simulink model "sm_rack_and_pinion_assembly_testrig"  (R2026a)
settings: Solver=ode23t  MaxStep=0.01  AbsTol=1e-4  EnableMultiTasking=on
undefined symbols (not defined in the file or in its folder): Local, Z
libraries: sm_lib x3, nesl_utility x2, Multibody_Parts_Lib x2
CloseFcn:
  | try,close(h1_sm_rack_and_pinion_assembly_testrig),end
  | clear h1_sm_rack_and_pinion_assembly_testrig
  | 
  | clear simlog_sm_rack_and_pinion_assembly_testrig
  | clear logsout_sm_rack_and_pinion_assembly_testrig
Description:
  | Rack and Pinion Assembly Testrig
  | 
  | Copyright 2014-2026 The MathWorks, Inc.
settings Model: Creator=smiller  LastModifiedBy=smiller
settings DataIOCC: SignalLoggingName=logsout_sm_rack_and_pinion_assembly_testrig
settings DebuggingCC: UnderspecifiedInitializationDetection=Classic  PregeneratedLibrarySubsystemCodeDiagnostic=none
settings HardwareCC: ProdHWDeviceType=32-bit Generic
settings SimscapeCC: SimscapeNormalizeSystem=off  SimscapeNominalValues="[{\"value\":\"1\",\"unit\":\"A\"},{\"value\":\"1\",\"unit\":\"bar\"},{\"value\":\"1\",\"unit\":\"cm^2\"},{\"value\":\"1\",\"unit\":\"cm^3/s\"},{\"value\":\"1\",\"unit\":\"kJ/kg\"},{\"value\":\"1\",\"unit\":\"kW\"},{\"value\":\"1\",\"unit\":\"l\"},{\"value\":\"1\",\"unit\":\"N\"},{\"value\":\"1\",\"unit\":\"N*m\"},{\"value\":\"1\",\"unit\":\"V\"}]"  SimscapeLogSimulationStatistics=on  SimscapeLogName=simlog_sm_rack_and_pinion_assembly_testrig
settings ConfigurationSet: Description=SimMechanics 2G
settings ExplorerConfigSet: InternalSimMechanicsExplorerSettings="<ExplorerConfiguration><canonicalview>default</canonicalview><AnimationSetting><BasePlaybackSpeed>1.0</BasePlaybackSpeed><PlaybackSpeedFactor>0.25</PlaybackSpeedFactor></AnimationSetting><TilePanel><TileInfo><Tiles Columns=\"1\" Count=\"1\" Rows=\"1\"><Column Left=\"2\" Weight=\"1\"/><Column Left=\"655\"/><Row Top=\"2\" Weight=\"1\"/><Row Top=\"641\"/><Tile Height=\"1\" Width=\"1\" X=\"0\" Y=\"0\"/></Tiles></TileInfo><SceneInfo><SceneViewer><BGColor><R>1</R><G>1</G><B>1</B></BGColor><Camera><DoPerspective>off</DoPerspective><Position><X>-1.4737661376785469</X><Y>0.83781885551971791</Y><Z>1.1253265827967358</Z></Position><Center><X>0.02566190273717369</X><Y>0.18460641908010048</Y><Z>-0.0024121521875122565</Z></Center><Up><X>0.24453438478606104</X><Y>0.94396980972908617</Y><Z>-0.22163919548973215</Z></Up><ViewLimDist>1</ViewLimDist><YLim>0.48982843392812059</YLim><XLim>0.50071351023763433</XLim></Camera></SceneViewer></SceneInfo></TilePanel><MechEditorPanel><Cameras/><GfxPanelCameraMap/><VideoCreator><PlaybackSpeedRatio>1.0</PlaybackSpeedRatio><FrameRate>30</FrameRate><VideoFormat>Motion JPEG AVI</VideoFormat><FrameSize>auto</FrameSize></VideoCreator></MechEditorPanel></ExplorerConfiguration>"

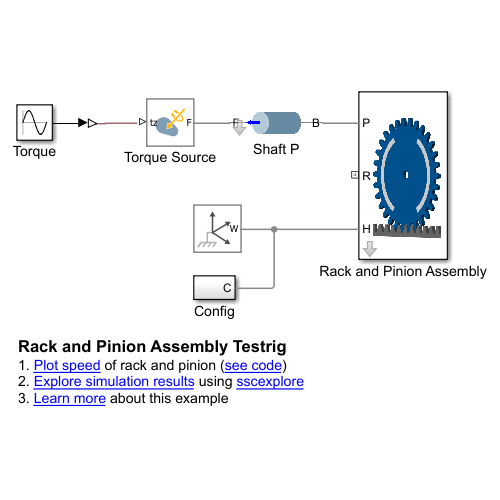
[thumbnail: Simulink's stored preview of the top-level diagram]
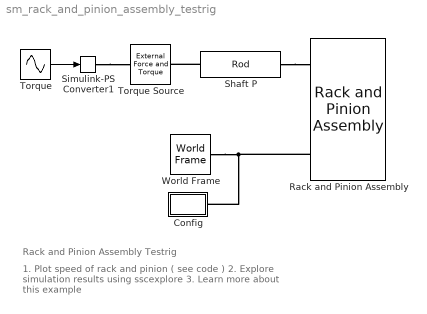
== system sm_rack_and_pinion_assembly_testrig ==
  note: Rack and Pinion Assembly Testrig
  note: 1. Plot speed of rack and pinion ( see code )
      | 2. Explore simulation results using sscexplore
      | 3. Learn more about this example
  Config : Subsystem
  Rack and Pinion Assembly : Multibody_Parts_Lib/Gears/Assemblies/Rack and Pinion Assembly  Tag=PublishSubsystem  pinion_pd_asy=0.5  pinion_nt_asy=30  pinion_th_asy=0.02  pinion_rh_asy=0.02  pinion_rho_asy=7000  pinion_clr_asy=[0 0.4 0.7]  pinion_opc_asy=1  p_popup_ad_dd=Default  pinion_ad_asy=0.5/30  pinion_dd_asy=1.157*0.5/30  pinion_visc_frict_asy=0  p_popup_markings=Two  p_mark_radius_range=[0.7 0.8]  p_mark_angle_range=120  p_mark_color=[1 1 1]  rack_tp_asy=0.052  rack_nt_asy=29  rack_tb_asy=0.02  rack_th_asy=0.02  rack_rho_asy=7000  rack_clr_asy=[0.5 0.5 0.5]  rack_opc_asy=1  r_popup_ad_dd=Default  rack_ad_asy=0.052/3.1416  rack_dd_asy=1.157*(0.052/3.1416)  rack_visc_frict_asy=0
      settings: SourceProductName=Simscape Multibody Parts Library
  Shaft P : Multibody_Parts_Lib/Basic/Rod  rod_rad=0.02  rod_len=0.3  rod_rho=7000  rod_color=[0 0.4 0.7]  rod_opc=1  popup_zori=Local +Z  popup_markings=None  mark_radius_range=[0.5 1.01]  mark_length_range=1.005  mark_angle_range=30  mark_color=[1 1 1]
      settings: SourceProductName=Simscape Multibody Parts Library
  Simulink-PS Converter1 : nesl_utility/Simulink-PS Converter  PhysicalDomain=network_engine_domain  SubClassName=ps_input  LeftPortType=input  RightPortType=output  PseudoPeriodic=off  Frequencies=[]  NoiseDistribution=none  NoiseParameters=[]  Unit=1  AffineConversion=off  FilteringAndDerivatives=zero  SimscapeFilterOrder=1  InputFilterTimeConstant=0.001  UdotUserProvided=1
  Torque : Sin  Amplitude=10  Frequency=pi  Phase=pi/2  SampleTime=0
  Torque Source : sm_lib/Forces and Torques/External Force and Torque  EnableForceX=off  EnableForceY=off  EnableForceZ=off  EnableForce=off  ForceResolutionFrame=AttachedFrame  EnableTorqueX=off  EnableTorqueY=off  EnableTorqueZ=on  EnableTorque=off  TorqueResolutionFrame=AttachedFrame
  World Frame : sm_lib/Frames and Transforms/World Frame
  wires:
  Torque/1 -> Simulink-PS Converter1/1
  connections:
  World Frame/RConn1 -- Rack and Pinion Assembly/LConn3 -- Config/LConn1
  Shaft P/LConn1 -- Rack and Pinion Assembly/LConn1
  Simulink-PS Converter1/RConn1 -- Torque Source/LConn1
  Shaft P/RConn1 -- Torque Source/RConn1

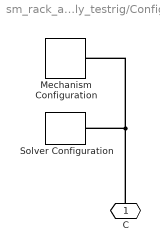
== system sm_rack_and_pinion_assembly_testrig/Config ==
  Mechanism Configuration : sm_lib/Utilities/Mechanism Configuration  UniformGravity=Constant  GravityVector=[0 -9.81 0]  GravityVectorUnits=m/s^2  LinearizationDelta=0.001  JointModeTransitionNonlinearIterations=2
  Solver Configuration : nesl_utility/Solver Configuration  PhysicalDomain=network_engine_domain  SubClassName=solver  LeftPortType=input  RightPortType=generic  Tones=[]  Harmonics=[]  SimulateNoise=off  Profile=off  UseLocalSampling=off  EnableSwitchedLinearOptims=on  FrequencyDomain=off  UseCCode=off  RelTol=0.001  AbsTol=1e-06  MinStep=1e-09  ToWorkspace=off  RevertToSquareIcSolve=off  NumHomotopyIterations=100  PhasorMode=off  PhasorModeNumHarmonics=1  ConsistencySolver=NEWTON_FTOL  CanonicalOrdering=UNORDERED  OptimizeIntermediates=UNOPTIMIZED  IndexReductionMethod=DerivativeReplacement  DoDC=off  ResidualTolerance=1e-09  ConsistencyTolSource=GLOBAL  ConsistencyAbsTol=0.001  ConsistencyRelTol=0.001  ConsistencyTolFactor=0.001  UseLocalSolver=off  LocalSolverChoice=NE_BACKWARD_EULER_ADVANCER  ResolveIndetEquations=on  FunctionEvalNumThread=1  LocalSolverSampleTime=0.001  DoFixedCost=off  MaxNonlinIter=3  MaxModeIter=2  ComputeImpulses=off  ImpulseIterations=2  LinearAlgebra=Sparse  LinearAlgebraNumThread=0  EquationFormulation=NE_TIME_EF  DelaysMemoryBudget=1024  AutomaticFiltering=on  FilteringTimeConstant=0.001  PartitionStorageMethod=AS_NEEDED  PartitionMemoryBudget=1024  PartitionMethod=FAST  MultibodyUseLocalSolver=off  MultibodyLocalSolverChoice=ODE1  MultibodyLocalSolverSampleTime=0.001
  C : PMIOPort  Side=Left
  connections:
  Mechanism Configuration/RConn1 -- C/RConn1 -- Solver Configuration/RConn1
